simulink model "euler2_NF"  (R2024b)
settings: Solver=FixedStepAuto  StartTime=0.0  StopTime=50  FixedStep=0.01  RelTol=1e-3
libraries: matrix_library x2, aerolibutil x2
settings Model: Creator=dr.gerardocastanon  LastModifiedBy=dr.gerardocastanon

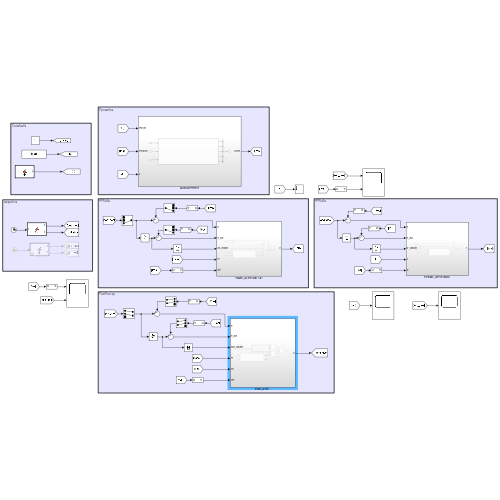
[thumbnail: Simulink's stored preview of the top-level diagram]
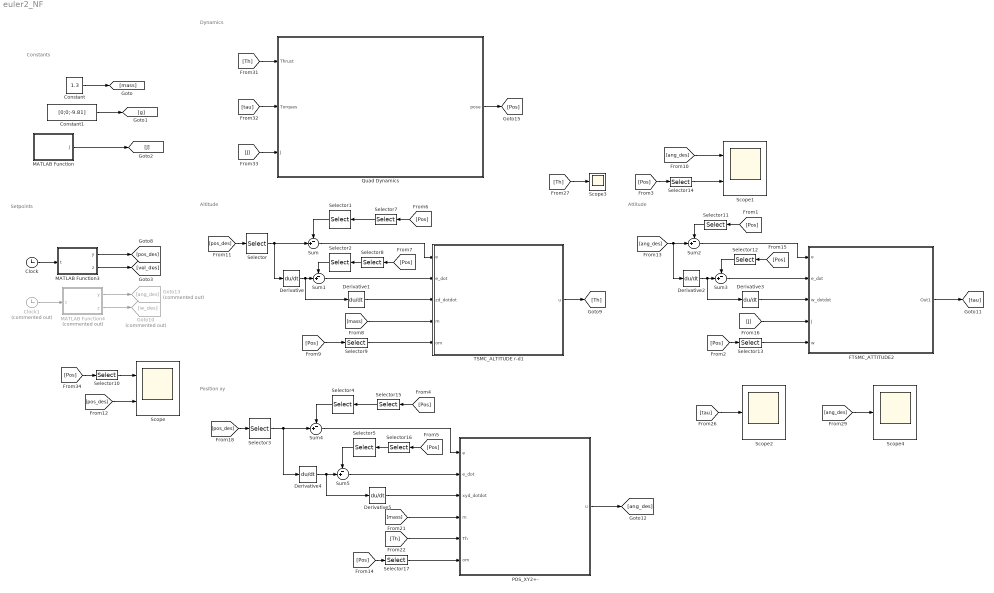
== system euler2_NF ==
  note: Constants
  note: Altitude
  note: Position xy
  note: Attitude
  note: Setpoints
  note: Dynamics
  Clock : Clock
  Clock1 : Clock  Commented=on
  Constant : Constant  Value=1.3
  Constant1 : Constant  Value=[0;0;-9.81]
  Derivative{,1..5} (6 alike) : Derivative
  FTSMC_ATTITUDE2 : Subsystem
  Goto10 : Goto  Commented=on  GotoTag=w_des
  Goto13 : Goto  Commented=on  GotoTag=ang_des
  MATLAB Function : MATLAB Function  TreatAsAtomicUnit=on
  MATLAB Function3 : MATLAB Function  TreatAsAtomicUnit=on
  MATLAB Function4 : MATLAB Function  Commented=on  TreatAsAtomicUnit=on
  POS_XY2+- : Subsystem
  Quad Dynamics : Subsystem
  Scope : Scope  NumInputPorts=2
  Scope1 : Scope  NumInputPorts=2
  Scope2 : Scope
  Scope3 : Scope
  Scope4 : Scope
  Selector : Selector  InputPortWidth=3  IndexOptions=Index vector (dialog)  Indices=[3]  OutputSizes=1
  Selector1 : Selector  InputPortWidth=3  IndexOptions=Index vector (dialog)  Indices=[3]  OutputSizes=1
  Selector10 : Selector  InputPortWidth=15  IndexOptions=Starting index (dialog)  Indices=[1]  OutputSizes=3
  Selector11 : Selector  InputPortWidth=15  IndexOptions=Starting index (dialog)  Indices=[10]  OutputSizes=3
  Selector12 : Selector  InputPortWidth=15  IndexOptions=Starting index (dialog)  Indices=[13]  OutputSizes=3
  Selector13 : Selector  InputPortWidth=15  IndexOptions=Starting index (dialog)  Indices=[13]  OutputSizes=3
  Selector14 : Selector  InputPortWidth=15  IndexOptions=Starting index (dialog)  Indices=[10]  OutputSizes=3
  Selector15 : Selector  InputPortWidth=15  IndexOptions=Starting index (dialog)  Indices=[1]  OutputSizes=3
  Selector16 : Selector  InputPortWidth=15  IndexOptions=Starting index (dialog)  Indices=[4]  OutputSizes=3
  Selector17 : Selector  InputPortWidth=15  IndexOptions=Starting index (dialog)  Indices=[13]  OutputSizes=3
  Selector2 : Selector  InputPortWidth=3  IndexOptions=Index vector (dialog)  Indices=[3]  OutputSizes=1
  Selector3 : Selector  InputPortWidth=3  IndexOptions=Index vector (dialog)  Indices=[1 2]  OutputSizes=1
  Selector4 : Selector  InputPortWidth=3  IndexOptions=Index vector (dialog)  Indices=[1 2]  OutputSizes=1
  Selector5 : Selector  InputPortWidth=3  IndexOptions=Index vector (dialog)  Indices=[1 2]  OutputSizes=1
  Selector7 : Selector  InputPortWidth=15  IndexOptions=Starting index (dialog)  Indices=[1]  OutputSizes=3
  Selector8 : Selector  InputPortWidth=15  IndexOptions=Starting index (dialog)  Indices=[4]  OutputSizes=3
  Selector9 : Selector  InputPortWidth=15  IndexOptions=Starting index (dialog)  Indices=[10]  OutputSizes=3
  Sum{,1..5} (6 alike) : Sum  Inputs=-+|
  TSMC_ALTITUDE r-d1 : Subsystem
  wires:
  Constant1/1 -> [g]
  Constant/1 -> [mass]
  MATLAB Function/1(J) -> [J]
  TSMC_ALTITUDE r-d1/1(u) -> [Th]
  Sum/1 -> TSMC_ALTITUDE r-d1/1(e)
  Sum1/1 -> TSMC_ALTITUDE r-d1/2(e_dot)
  Derivative1/1 -> TSMC_ALTITUDE r-d1/3(zd_dotdot)
  [mass] -> TSMC_ALTITUDE r-d1/4(m)
  [Pos] -> Selector9/1
  Selector1/1 -> Sum/1
  [Pos] -> Selector8/1
  Selector2/1 -> Sum1/1
  Selector10/1 -> Scope/1
  Clock/1 -> MATLAB Function3/1(t)
  MATLAB Function3/1(y) -> [pos_des]
  Selector/1 -> Derivative/1, Sum/2
  [pos_des] -> Scope/2
  [pos_des] -> Selector/1
  [ang_des] -> Derivative2/1, Sum2/2
  Selector11/1 -> Sum2/1
  Sum2/1 -> FTSMC_ATTITUDE2/1(e)
  Sum3/1 -> FTSMC_ATTITUDE2/2(e_dot)
  Derivative3/1 -> FTSMC_ATTITUDE2/3(w_dotdot)
  [J] -> FTSMC_ATTITUDE2/4(J)
  FTSMC_ATTITUDE2/1(Out1) -> [tau]
  Selector13/1 -> FTSMC_ATTITUDE2/5(w)
  Selector4/1 -> Sum4/1
  [pos_des] -> Selector3/1
  Selector3/1 -> Sum4/2, Derivative4/1
  Derivative4/1 -> Derivative5/1, Sum5/2
  Selector5/1 -> Sum5/1
  Selector15/1 -> Selector4/1
  Sum5/1 -> POS_XY2+-/2(e_dot)
  Sum4/1 -> POS_XY2+-/1(e)
  [mass] -> POS_XY2+-/4(m)
  [Th] -> POS_XY2+-/5(Th)
  MATLAB Function4/1(y) -> Goto13/1
  Clock1/1 -> MATLAB Function4/1(t)
  [ang_des] -> Scope1/1
  Selector14/1 -> Scope1/2
  [Th] -> Scope3/1
  Selector17/1 -> POS_XY2+-/6(om)
  [ang_des] -> Scope4/1
  POS_XY2+-/1(u) -> [ang_des]
  MATLAB Function3/2(z) -> [vel_des]
  MATLAB Function4/2(z) -> Goto10/1
  Derivative5/1 -> POS_XY2+-/3(xyd_dotdot)
  Derivative2/1 -> Sum3/2, Derivative3/1
  [tau] -> Scope2/1
  Derivative/1 -> Derivative1/1, Sum1/2
  Quad Dynamics/1(pose) -> [Pos]
  [Pos] -> Selector7/1
  Selector7/1 -> Selector1/1
  Selector8/1 -> Selector2/1
  [tau] -> Quad Dynamics/2(Torques)
  [Th] -> Quad Dynamics/1(Thrust)
  [J] -> Quad Dynamics/3(J)
  Selector9/1 -> TSMC_ALTITUDE r-d1/5(om)
  [Pos] -> Selector10/1
  [Pos] -> Selector11/1
  Selector12/1 -> Sum3/1
  [Pos] -> Selector12/1
  [Pos] -> Selector13/1
  [Pos] -> Selector14/1
  [Pos] -> Selector15/1
  [Pos] -> Selector16/1
  Selector16/1 -> Selector5/1
  [Pos] -> Selector17/1

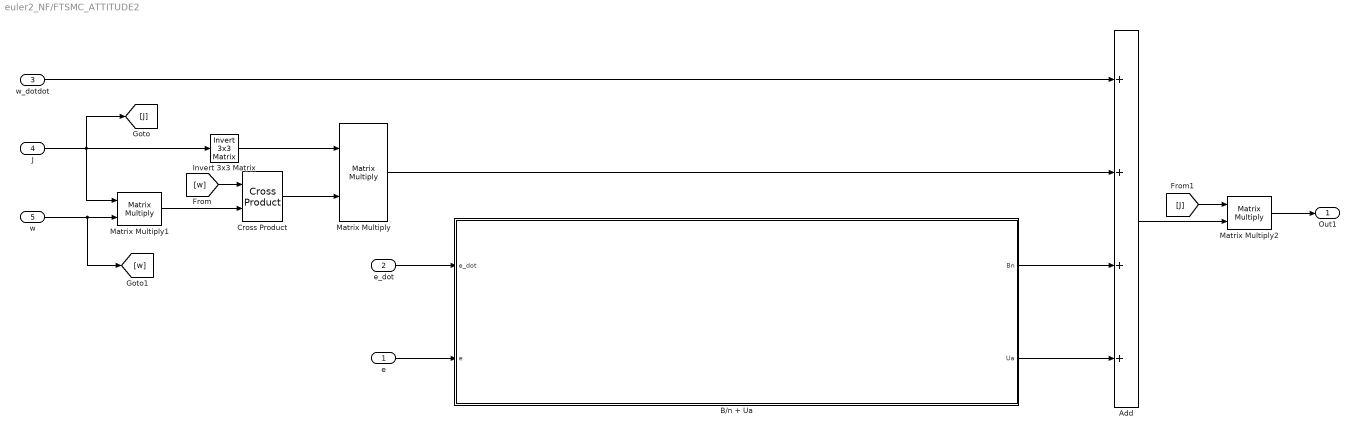
== system euler2_NF/FTSMC_ATTITUDE2 ==
  e : Inport
  e_dot : Inport  Port=2
  w_dotdot : Inport  Port=3
  J : Inport  Port=4
  w : Inport  Port=5
  Add : Sum  Inputs=++++
  B/n + Ua : Subsystem
  Cross Product : matrix_library/Cross Product
  Invert 3x3 Matrix : aerolibutil/Invert  3x3 Matrix
  Matrix Multiply : Product  Multiplication=Matrix(*)
  Matrix Multiply1 : Product  Multiplication=Matrix(*)
  Matrix Multiply2 : Product  Multiplication=Matrix(*)
  Out1 : Outport
  wires:
  J/1 -> [J], Matrix Multiply1/1, Invert 3x3 Matrix/1
  Invert 3x3 Matrix/1 -> Matrix Multiply/1
  Cross Product/1 -> Matrix Multiply/2
  Matrix Multiply1/1 -> Cross Product/2
  w/1 -> [w], Matrix Multiply1/2
  [w] -> Cross Product/1
  w_dotdot/1 -> Add/1
  Matrix Multiply/1 -> Add/2
  Add/1 -> Matrix Multiply2/2
  Matrix Multiply2/1 -> Out1/1
  [J] -> Matrix Multiply2/1
  B/n + Ua/1(Bn) -> Add/3
  B/n + Ua/2(Ua) -> Add/4
  e_dot/1 -> B/n + Ua/1(e_dot)
  e/1 -> B/n + Ua/2(e)

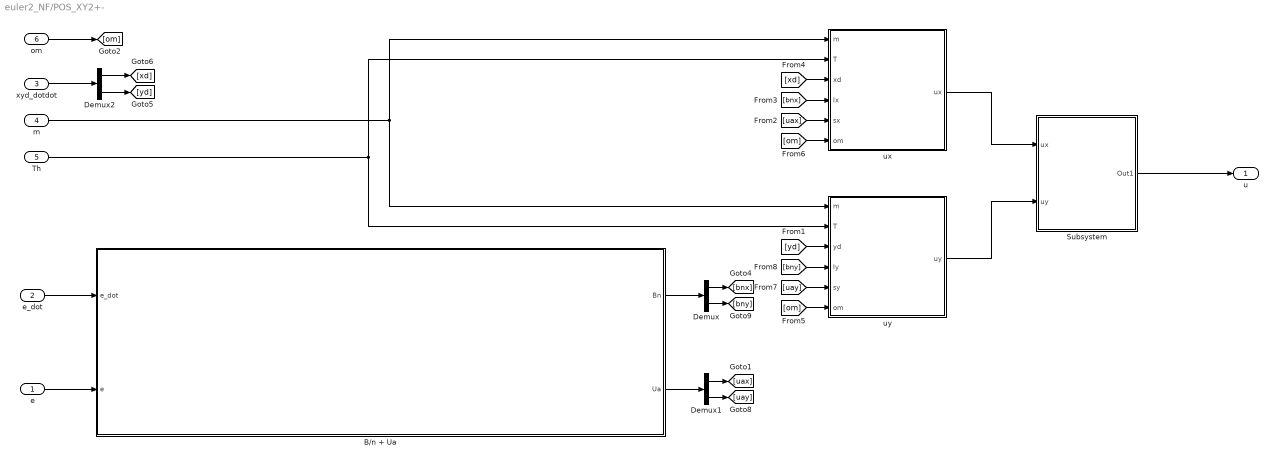
== system euler2_NF/POS_XY2+- ==
  e : Inport
  e_dot : Inport  Port=2
  xyd_dotdot : Inport  Port=3
  m : Inport  Port=4
  Th : Inport  Port=5
  om : Inport  Port=6
  B/n + Ua : Subsystem
  Demux : Demux  Outputs=2
  Demux1 : Demux  Outputs=2
  Demux2 : Demux  Outputs=2
  Subsystem : Subsystem
  ux : Subsystem
  uy : Subsystem
  u : Outport
  wires:
  Demux1/1 -> [uax]
  Demux/1 -> [bnx]
  xyd_dotdot/1 -> Demux2/1
  Demux2/1 -> [xd]
  Demux2/2 -> [yd]
  m/1 -> ux/1(m), uy/1(m)
  [yd] -> uy/3(yd)
  [uax] -> ux/5(sx)
  [bnx] -> ux/4(lx)
  [xd] -> ux/3(xd)
  om/1 -> [om]
  [om] -> uy/6(om)
  [om] -> ux/6(om)
  Subsystem/1(Out1) -> u/1
  ux/1(ux) -> Subsystem/1(ux)
  uy/1(uy) -> Subsystem/2(uy)
  Th/1 -> ux/2(T), uy/2(T)
  Demux1/2 -> [uay]
  [uay] -> uy/5(sy)
  Demux/2 -> [bny]
  [bny] -> uy/4(ly)
  e_dot/1 -> B/n + Ua/1(e_dot)
  e/1 -> B/n + Ua/2(e)
  B/n + Ua/2(Ua) -> Demux1/1
  B/n + Ua/1(Bn) -> Demux/1

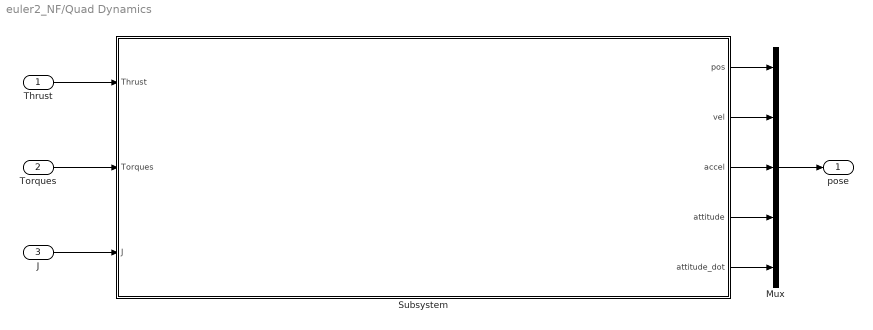
== system euler2_NF/Quad Dynamics ==
  Thrust : Inport
  Torques : Inport  Port=2
  J : Inport  Port=3
  Mux : Mux  Inputs=5
  Subsystem : Subsystem
  pose : Outport
  wires:
  Subsystem/1(pos) -> Mux/1
  Subsystem/2(vel) -> Mux/2
  Subsystem/3(accel) -> Mux/3
  Subsystem/4(attitude) -> Mux/4
  Subsystem/5(attitude_dot) -> Mux/5
  Thrust/1 -> Subsystem/1(Thrust)
  Torques/1 -> Subsystem/2(Torques)
  Mux/1 -> pose/1
  J/1 -> Subsystem/3(J)

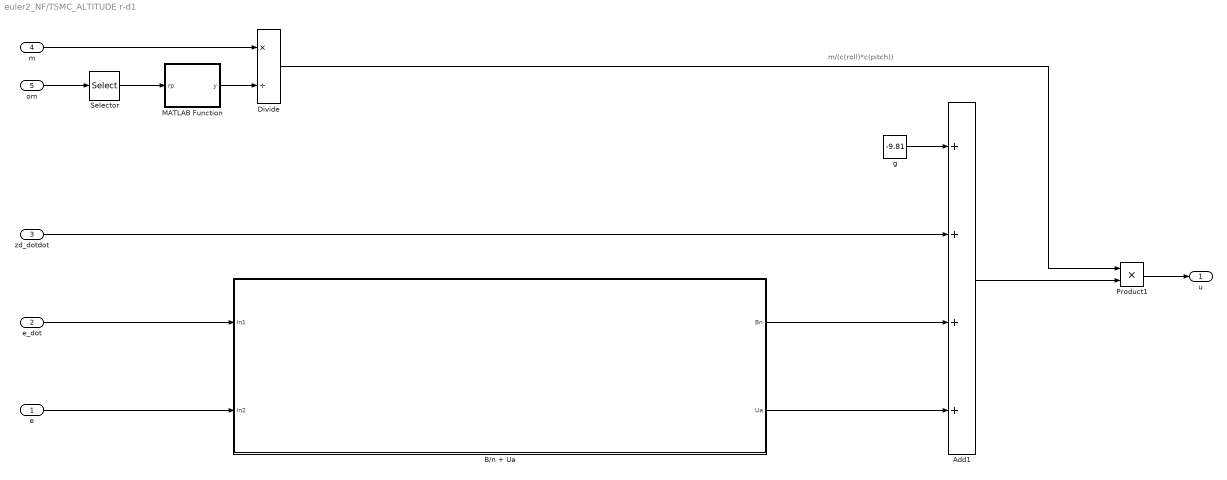
== system euler2_NF/TSMC_ALTITUDE r-d1 ==
  note: m/(c(roll)*c(pitch))
  e : Inport
  e_dot : Inport  Port=2
  zd_dotdot : Inport  Port=3
  m : Inport  Port=4
  om : Inport  Port=5
  Add1 : Sum  Inputs=++++
  B/n + Ua : Subsystem
  Divide : Product  Inputs=*/
  MATLAB Function : MATLAB Function  TreatAsAtomicUnit=on
  Product1 : Product
  Selector : Selector  InputPortWidth=3  IndexOptions=Index vector (dialog)  Indices=[1 2]  OutputSizes=1
  g : Constant  Value=-9.81
  u : Outport
  wires:
  Selector/1 -> MATLAB Function/1(rp)
  MATLAB Function/1(y) -> Divide/2
  m/1 -> Divide/1
  g/1 -> Add1/1
  Divide/1 -> Product1/1
  om/1 -> Selector/1
  Product1/1 -> u/1
  zd_dotdot/1 -> Add1/2
  Add1/1 -> Product1/2
  e_dot/1 -> B/n + Ua/1(In1)
  e/1 -> B/n + Ua/2(In2)
  B/n + Ua/1(Bn) -> Add1/3
  B/n + Ua/2(Ua) -> Add1/4

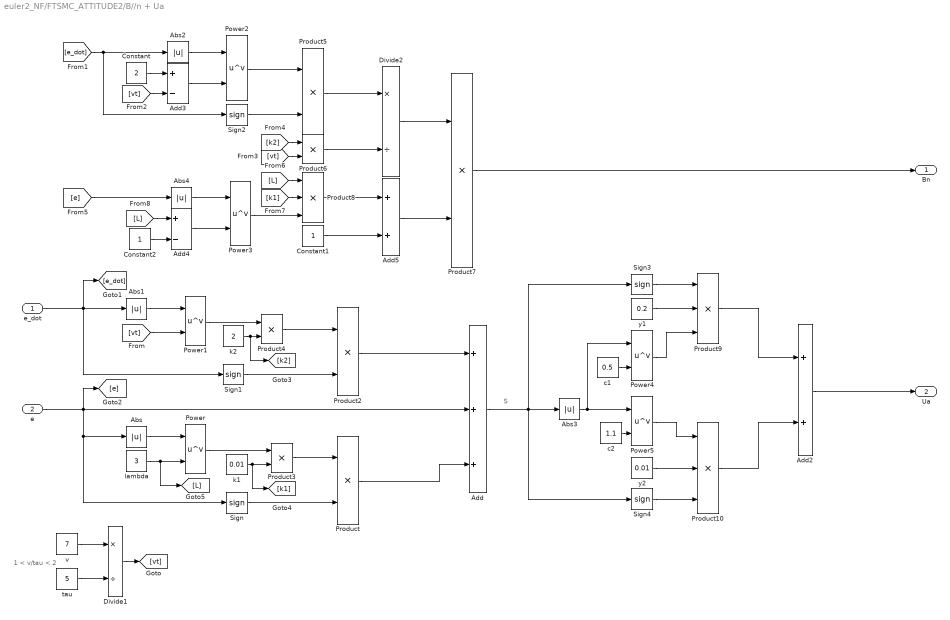
== system euler2_NF/FTSMC_ATTITUDE2/B//n + Ua ==
  note: S
  note: 1 < v/tau < 2
  e_dot : Inport
  e : Inport  Port=2
  Abs{,1..4} (5 alike) : Abs  SaturateOnIntegerOverflow=off
  Add : Sum  Inputs=+++
  Add2 : Sum
  Add3 : Sum  Inputs=+-
  Add4 : Sum  Inputs=+-
  Add5 : Sum
  Constant : Constant  Value=2
  Constant1 : Constant
  Constant2 : Constant
  Divide1 : Product  Inputs=*/
  Divide2 : Product  Inputs=*/
  Power{,1..5} (6 alike) : Math  Operator=pow
  Product{,2..7} (7 alike) : Product
  Product10 : Product  Inputs=3
  Product8 : Product  Inputs=3
  Product9 : Product  Inputs=3
  Sign{,1..4} (5 alike) : Signum
  c1 : Constant  Value=0.5
  c2 : Constant  Value=1.1
  k1 : Constant  Value=0.01
  k2 : Constant  Value=2
  lambda : Constant  Value=3
  tau : Constant  Value=5
  v : Constant  Value=7
  y1 : Constant  Value=0.2
  y2 : Constant  Value=0.01
  Bn : Outport
  Ua : Outport  Port=2
  wires:
  y1/1 -> Product9/2
  Constant1/1 -> Add5/2
  [k2] -> Product6/1
  Power3/1 -> Product8/3
  Product5/1 -> Divide2/1
  Abs3/1 -> Power4/1, Power5/1
  c2/1 -> Power5/2
  Product6/1 -> Divide2/2
  k1/1 -> Product3/2, [k1]
  tau/1 -> Divide1/2
  lambda/1 -> [L], Power/2
  [vt] -> Power1/2
  [vt] -> Product6/2
  [e_dot] -> Sign2/1, Abs2/1
  Power1/1 -> Product4/1
  Sign1/1 -> Product2/2
  Add4/1 -> Power3/2
  [k1] -> Product8/2
  Product/1 -> Add/3
  e/1 -> [e], Abs/1, Sign/1, Add/2
  Constant2/1 -> Add4/2
  Product9/1 -> Add2/1
  Add/1 -> Sign4/1, Sign3/1, Abs3/1
  v/1 -> Divide1/1
  Sign/1 -> Product/2
  c1/1 -> Power4/2
  k2/1 -> [k2], Product4/2
  Sign3/1 -> Product9/1
  Sign2/1 -> Product5/2
  Add3/1 -> Power2/2
  Power2/1 -> Product5/1
  Product10/1 -> Add2/2
  Abs2/1 -> Power2/1
  Abs/1 -> Power/1
  Constant/1 -> Add3/1
  [vt] -> Add3/2
  [L] -> Add4/1
  Add2/1 -> Ua/1
  Abs1/1 -> Power1/1
  [L] -> Product8/1
  e_dot/1 -> [e_dot], Abs1/1, Sign1/1
  Add5/1 -> Product7/2
  [e] -> Abs4/1
  Divide2/1 -> Product7/1
  Power5/1 -> Product10/1
  Product3/1 -> Product/1
  Power/1 -> Product3/1
  Power4/1 -> Product9/3
  Sign4/1 -> Product10/3
  Product8/1 -> Add5/1
  y2/1 -> Product10/2
  Product2/1 -> Add/1
  Abs4/1 -> Power3/1
  Product4/1 -> Product2/1
  Divide1/1 -> [vt]
  Product7/1 -> Bn/1

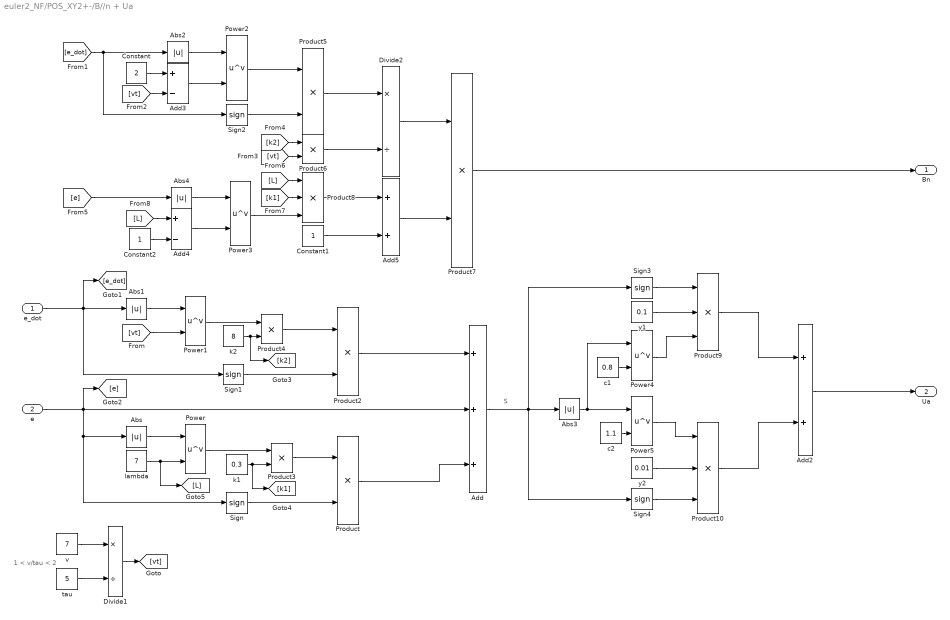
== system euler2_NF/POS_XY2+-/B//n + Ua ==
  note: S
  note: 1 < v/tau < 2
  e_dot : Inport
  e : Inport  Port=2
  Abs{,1..4} (5 alike) : Abs  SaturateOnIntegerOverflow=off
  Add : Sum  Inputs=+++
  Add2 : Sum
  Add3 : Sum  Inputs=+-
  Add4 : Sum  Inputs=+-
  Add5 : Sum
  Constant : Constant  Value=2
  Constant1 : Constant
  Constant2 : Constant
  Divide1 : Product  Inputs=*/
  Divide2 : Product  Inputs=*/
  Power{,1..5} (6 alike) : Math  Operator=pow
  Product{,2..7} (7 alike) : Product
  Product10 : Product  Inputs=3
  Product8 : Product  Inputs=3
  Product9 : Product  Inputs=3
  Sign{,1..4} (5 alike) : Signum
  c1 : Constant  Value=0.8
  c2 : Constant  Value=1.1
  k1 : Constant  Value=0.3
  k2 : Constant  Value=8
  lambda : Constant  Value=7
  tau : Constant  Value=5
  v : Constant  Value=7
  y1 : Constant  Value=0.1
  y2 : Constant  Value=0.01
  Bn : Outport
  Ua : Outport  Port=2
  wires:
  y1/1 -> Product9/2
  Constant1/1 -> Add5/2
  [k2] -> Product6/1
  Power3/1 -> Product8/3
  Product5/1 -> Divide2/1
  Abs3/1 -> Power4/1, Power5/1
  c2/1 -> Power5/2
  Product6/1 -> Divide2/2
  k1/1 -> Product3/2, [k1]
  tau/1 -> Divide1/2
  lambda/1 -> [L], Power/2
  [vt] -> Power1/2
  [vt] -> Product6/2
  [e_dot] -> Sign2/1, Abs2/1
  Power1/1 -> Product4/1
  Sign1/1 -> Product2/2
  Add4/1 -> Power3/2
  [k1] -> Product8/2
  Product/1 -> Add/3
  e/1 -> [e], Abs/1, Sign/1, Add/2
  Constant2/1 -> Add4/2
  Product9/1 -> Add2/1
  Add/1 -> Sign3/1, Sign4/1, Abs3/1
  v/1 -> Divide1/1
  Sign/1 -> Product/2
  c1/1 -> Power4/2
  k2/1 -> [k2], Product4/2
  Sign3/1 -> Product9/1
  Sign2/1 -> Product5/2
  Add3/1 -> Power2/2
  Power2/1 -> Product5/1
  Product10/1 -> Add2/2
  Abs2/1 -> Power2/1
  Abs/1 -> Power/1
  Constant/1 -> Add3/1
  [vt] -> Add3/2
  [L] -> Add4/1
  Add2/1 -> Ua/1
  Abs1/1 -> Power1/1
  [L] -> Product8/1
  e_dot/1 -> [e_dot], Abs1/1, Sign1/1
  Add5/1 -> Product7/2
  [e] -> Abs4/1
  Divide2/1 -> Product7/1
  Power5/1 -> Product10/1
  Product3/1 -> Product/1
  Power/1 -> Product3/1
  Power4/1 -> Product9/3
  Sign4/1 -> Product10/3
  Product8/1 -> Add5/1
  y2/1 -> Product10/2
  Product2/1 -> Add/1
  Abs4/1 -> Power3/1
  Product4/1 -> Product2/1
  Divide1/1 -> [vt]
  Product7/1 -> Bn/1

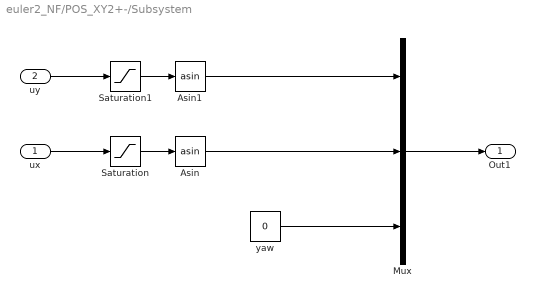
== system euler2_NF/POS_XY2+-/Subsystem ==
  ux : Inport
  uy : Inport  Port=2
  Asin : Trigonometry  Operator=asin
  Asin1 : Trigonometry  Operator=asin
  Mux : Mux  Inputs=3
  Saturation : Saturate  UpperLimit=1  LowerLimit=-1  ZeroCross=off
  Saturation1 : Saturate  UpperLimit=1  LowerLimit=-1  ZeroCross=off
  yaw : Constant  Value=0
  Out1 : Outport
  wires:
  ux/1 -> Saturation/1
  uy/1 -> Saturation1/1
  Asin1/1 -> Mux/1
  Asin/1 -> Mux/2
  yaw/1 -> Mux/3
  Mux/1 -> Out1/1
  Saturation/1 -> Asin/1
  Saturation1/1 -> Asin1/1

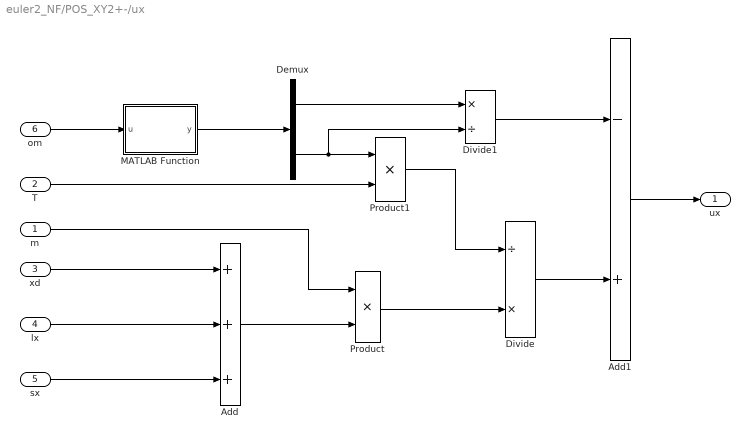
== system euler2_NF/POS_XY2+-/ux ==
  m : Inport
  T : Inport  Port=2
  xd : Inport  Port=3
  lx : Inport  Port=4
  sx : Inport  Port=5
  om : Inport  Port=6
  Add : Sum  Inputs=+++
  Add1 : Sum  Inputs=-+
  Demux : Demux  Outputs=2
  Divide : Product  Inputs=/*
  Divide1 : Product  Inputs=*/
  MATLAB Function : MATLAB Function  TreatAsAtomicUnit=on
  Product : Product
  Product1 : Product
  ux : Outport
  wires:
  xd/1 -> Add/1
  lx/1 -> Add/2
  Add/1 -> Product/2
  m/1 -> Product/1
  Product/1 -> Divide/2
  om/1 -> MATLAB Function/1(u)
  MATLAB Function/1(y) -> Demux/1
  Demux/2 -> Divide1/2, Product1/1
  T/1 -> Product1/2
  Product1/1 -> Divide/1
  Demux/1 -> Divide1/1
  Divide1/1 -> Add1/1
  Divide/1 -> Add1/2
  Add1/1 -> ux/1
  sx/1 -> Add/3

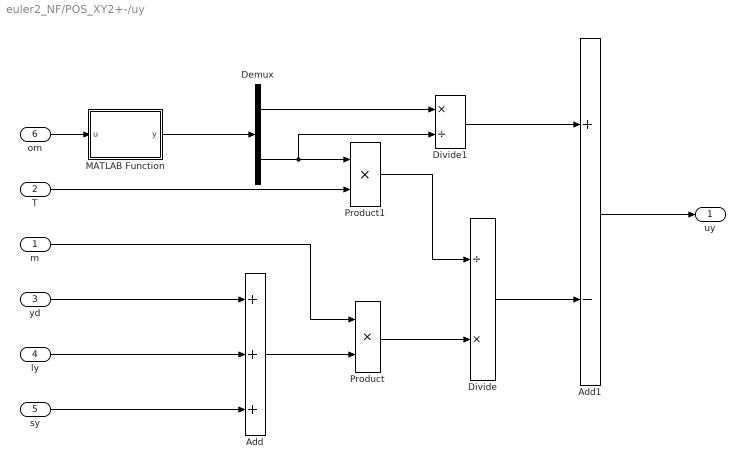
== system euler2_NF/POS_XY2+-/uy ==
  m : Inport
  T : Inport  Port=2
  yd : Inport  Port=3
  ly : Inport  Port=4
  sy : Inport  Port=5
  om : Inport  Port=6
  Add : Sum  Inputs=+++
  Add1 : Sum  Inputs=+-
  Demux : Demux  Outputs=2
  Divide : Product  Inputs=/*
  Divide1 : Product  Inputs=*/
  MATLAB Function : MATLAB Function  TreatAsAtomicUnit=on
  Product : Product
  Product1 : Product
  uy : Outport
  wires:
  om/1 -> MATLAB Function/1(u)
  yd/1 -> Add/1
  ly/1 -> Add/2
  sy/1 -> Add/3
  Add/1 -> Product/2
  m/1 -> Product/1
  MATLAB Function/1(y) -> Demux/1
  Divide1/1 -> Add1/1
  Demux/1 -> Divide1/1
  Demux/2 -> Divide1/2, Product1/1
  Add1/1 -> uy/1
  Product1/1 -> Divide/1
  T/1 -> Product1/2
  Product/1 -> Divide/2
  Divide/1 -> Add1/2

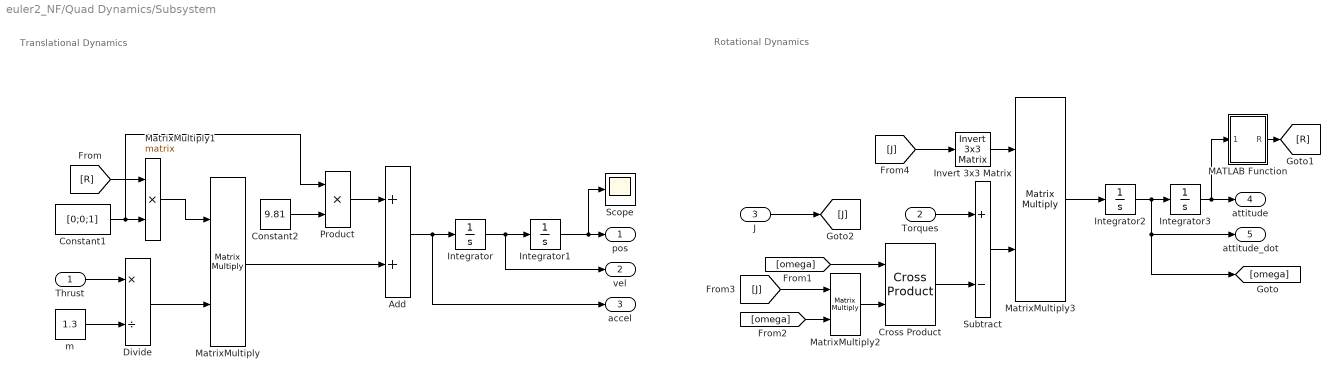
== system euler2_NF/Quad Dynamics/Subsystem ==
  note: Rotational Dynamics
  note: Translational Dynamics
  Thrust : Inport
  Torques : Inport  Port=2
  J : Inport  Port=3
  Add : Sum
  Constant1 : Constant  Value=[0;0;1]
  Constant2 : Constant  Value=9.81
  Cross Product : matrix_library/Cross Product
  Divide : Product  Inputs=*/
  Integrator{,1..3} (4 alike) : Integrator
  Invert 3x3 Matrix : aerolibutil/Invert  3x3 Matrix
  MATLAB Function : MATLAB Function  TreatAsAtomicUnit=on
  MatrixMultiply{,1..3} (4 alike) : Product  Multiplication=Matrix(*)
  Product : Product
  Scope : Scope
  Subtract : Sum  Inputs=+-
  m : Constant  Value=1.3
  pos : Outport
  vel : Outport  Port=2
  accel : Outport  Port=3
  attitude : Outport  Port=4
  attitude_dot : Outport  Port=5
  wires:
  m/1 -> Divide/2
  MatrixMultiply1/1 -> MatrixMultiply/1
  Integrator2/1 -> [omega], attitude_dot/1, Integrator3/1
  Constant2/1 -> Product/2
  Integrator1/1 -> Scope/1, pos/1
  Integrator/1 -> vel/1, Integrator1/1
  [J] -> Invert 3x3 Matrix/1
  [omega] -> Cross Product/1
  [J] -> MatrixMultiply2/1
  [omega] -> MatrixMultiply2/2
  Cross Product/1 -> Subtract/2
  Divide/1 -> MatrixMultiply/2
  Torques/1 -> Subtract/1
  [R] -> MatrixMultiply1/1
  MatrixMultiply/1 -> Add/2
  Integrator3/1 -> MATLAB Function/1(att), attitude/1
  MATLAB Function/1(R) -> [R]
  Constant1/1 -> Product/1, MatrixMultiply1/2
  MatrixMultiply3/1 -> Integrator2/1
  Add/1 -> accel/1, Integrator/1
  MatrixMultiply2/1 -> Cross Product/2
  Subtract/1 -> MatrixMultiply3/2
  Thrust/1 -> Divide/1
  Product/1 -> Add/1
  Invert 3x3 Matrix/1 -> MatrixMultiply3/1
  J/1 -> [J]

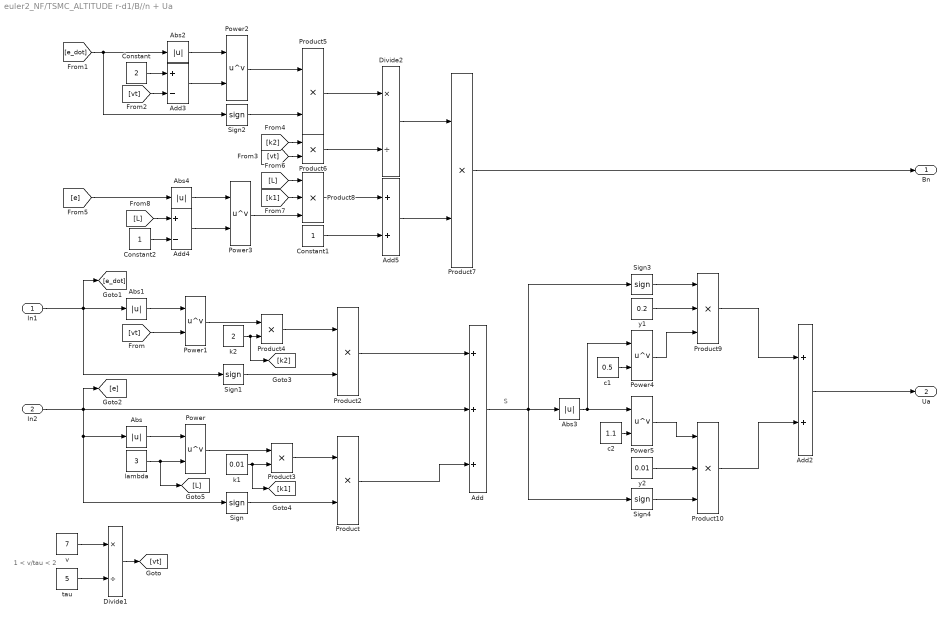
== system euler2_NF/TSMC_ALTITUDE r-d1/B//n + Ua ==
  note: S
  note: 1 < v/tau < 2
  In1 : Inport
  In2 : Inport  Port=2
  Abs{,1..4} (5 alike) : Abs  SaturateOnIntegerOverflow=off
  Add : Sum  Inputs=+++
  Add2 : Sum
  Add3 : Sum  Inputs=+-
  Add4 : Sum  Inputs=+-
  Add5 : Sum
  Constant : Constant  Value=2
  Constant1 : Constant
  Constant2 : Constant
  Divide1 : Product  Inputs=*/
  Divide2 : Product  Inputs=*/
  Power{,1..5} (6 alike) : Math  Operator=pow
  Product{,2..7} (7 alike) : Product
  Product10 : Product  Inputs=3
  Product8 : Product  Inputs=3
  Product9 : Product  Inputs=3
  Sign{,1..4} (5 alike) : Signum
  c1 : Constant  Value=0.5
  c2 : Constant  Value=1.1
  k1 : Constant  Value=0.01
  k2 : Constant  Value=2
  lambda : Constant  Value=3
  tau : Constant  Value=5
  v : Constant  Value=7
  y1 : Constant  Value=0.2
  y2 : Constant  Value=0.01
  Bn : Outport
  Ua : Outport  Port=2
  wires:
  y1/1 -> Product9/2
  Constant1/1 -> Add5/2
  [k2] -> Product6/1
  Power3/1 -> Product8/3
  Product5/1 -> Divide2/1
  Abs3/1 -> Power4/1, Power5/1
  c2/1 -> Power5/2
  Product6/1 -> Divide2/2
  k1/1 -> Product3/2, [k1]
  tau/1 -> Divide1/2
  lambda/1 -> [L], Power/2
  [vt] -> Power1/2
  [vt] -> Product6/2
  [e_dot] -> Sign2/1, Abs2/1
  Power1/1 -> Product4/1
  Sign1/1 -> Product2/2
  Add4/1 -> Power3/2
  [k1] -> Product8/2
  Product/1 -> Add/3
  In2/1 -> [e], Abs/1, Sign/1, Add/2
  Constant2/1 -> Add4/2
  Product9/1 -> Add2/1
  Add/1 -> Sign4/1, Sign3/1, Abs3/1
  v/1 -> Divide1/1
  Sign/1 -> Product/2
  c1/1 -> Power4/2
  k2/1 -> [k2], Product4/2
  Sign3/1 -> Product9/1
  Sign2/1 -> Product5/2
  Add3/1 -> Power2/2
  Power2/1 -> Product5/1
  Product10/1 -> Add2/2
  Abs2/1 -> Power2/1
  Abs/1 -> Power/1
  Constant/1 -> Add3/1
  [vt] -> Add3/2
  [L] -> Add4/1
  Add2/1 -> Ua/1
  Abs1/1 -> Power1/1
  [L] -> Product8/1
  In1/1 -> [e_dot], Abs1/1, Sign1/1
  Add5/1 -> Product7/2
  [e] -> Abs4/1
  Divide2/1 -> Product7/1
  Power5/1 -> Product10/1
  Product3/1 -> Product/1
  Power/1 -> Product3/1
  Power4/1 -> Product9/3
  Sign4/1 -> Product10/3
  Product8/1 -> Add5/1
  y2/1 -> Product10/2
  Product2/1 -> Add/1
  Abs4/1 -> Power3/1
  Product4/1 -> Product2/1
  Divide1/1 -> [vt]
  Product7/1 -> Bn/1

== matlab function euler2_NF/MATLAB Function3 ==
  data: t input; y output; z output
function [y,z]= fcn(t)

r = 0.1;

% y = [1;1;1];
y = [0.4;0.5;0.1];
% y = [r*cos(1*t) + r;r*sin(1*t);.1*t];
% y = [0;0;0.5];
z = [0;0;0];

== matlab function euler2_NF/TSMC_ALTITUDE r-d1/MATLAB Function ==
  data: rp input; y output
function y = fcn(rp)

y = cos(rp(1))*cos(rp(2));

== matlab function euler2_NF/MATLAB Function4 ==
  data: t input; y output; z output
function [y,z] = fcn(t)

r = 0.01;

% y = [r*cos(3*t);r*cos(2*t);0];
y = [0;0.5;1];
z = [0;0;0];

== matlab function euler2_NF/POS_XY2+-/ux/MATLAB Function ==
  data: u input; y output
function y = fcn(u)

y = [sin(u(1))*sin(u(3));cos(u(1))*cos(u(3))];

== matlab function euler2_NF/POS_XY2+-/uy/MATLAB Function ==
  data: u input; y output
function y = fcn(u)

y = [cos(u(1))*sin(u(2))*sin(u(3));cos(u(3))];

== matlab function euler2_NF/Quad Dynamics/Subsystem/MATLAB Function ==
  data: att input; R output
function R = fcn(att)
phi = att(1);
theta = att(2);
psi = att(3);

R = [
cos(psi)*cos(theta), cos(psi)*sin(theta)*sin(phi) - cos(phi)*sin(psi), cos(psi)*cos(phi)*sin(theta)+sin(phi)*sin(psi);
cos(theta)*sin(psi), sin(psi)*sin(phi)*sin(theta) + cos(phi)*cos(psi), sin(psi)*cos(phi)*sin(theta)-cos(psi)*sin(phi);
-sin(theta),cos(theta)*sin(phi), cos(phi)*cos(theta);
];

== matlab function euler2_NF/MATLAB Function ==
  data: J output
function J = fcn()

Jxx = 0.177;
Jyy = 0.177;
Jzz = 0.354; 

J = diag([Jxx,Jyy,Jzz]);
